simulink model "Esercizio6_sim"  (R2020b)
settings: Solver=VariableStepAuto  StartTime=0.0  StopTime=10.0  RelTol=1e-3
values from neighbouring files (symbols this model uses):
  Tc = 0.1    [Esercizio6.m]
settings Model: Creator=chiar  LastModifiedBy=chiar

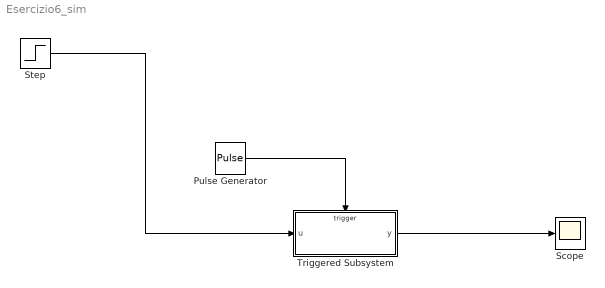
== system Esercizio6_sim ==
  Pulse Generator : DiscretePulseGenerator  PulseType=Time based  Period=Tc  PulseWidth=5
  Scope : Scope
  Step : Step  SampleTime=0
  Triggered Subsystem : Subsystem  TreatAsAtomicUnit=on
  wires:
  Pulse Generator/1 -> Triggered Subsystem/Trigger
  Step/1 -> Triggered Subsystem/1(u)
  Triggered Subsystem/1(y) -> Scope/1

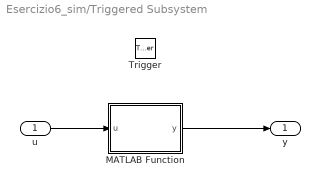
== system Esercizio6_sim/Triggered Subsystem ==
  u : Inport
  Trigger : TriggerPort  VariantControl=Variant
  MATLAB Function : MATLAB Function  TreatAsAtomicUnit=on
  y : Outport
  wires:
  u/1 -> MATLAB Function/1(u)
  MATLAB Function/1(y) -> y/1

== matlab function Esercizio6_sim/Triggered Subsystem/MATLAB Function ==
  data: u input; y output
function y = fcn(u)

%Scrivo l'equazione alle differenze che ho ricavato su quaderno

%Definisco le variabili PERSISTENT per renderle dotate di memoria e poter
%usare il valore per passi successivi

persistent ym1 ym2 um1 um2

%% 
%Definisco cosa succede all'istente 0

if isempty(ym1) %Se è vuota una delle variabili, inizializzo tutto a 0
    ym1=0;
    ym2=0;
    um1=0;
    um2=0;
end

%%
%Ricavo i coefficienti digitando cell2mat(sys.den)e sys.num per
%visualiazzare i coefficienti

%Per avere tanti decimali, digito formato long

%NB: metto solo i moduli dei coefficienti!

d1= 2.093337234759127;
d0= 1.094174283705210;
n2= 1.000000000000000 ;
n0= 1.002242763089924;


y = d1*ym1-d0*ym2+n2*u+n0*um2;

%%
%Preparo la funzione per l'istante successivo

ym2=ym1;
ym1=y;

um2=um1;
um1=u;
